simulink model "Filtri_Dinamici"  (R2022b)
settings: Solver=ode45  StartTime=0.0  StopTime=time_max  RelTol=1e-3
values from neighbouring files (symbols this model uses):
  b_omega_hat0 = [0;0;0]    [Main_Articolo.m]
  bias_accel = [bias_a_x; bias_a_y; bias_a_z]    [Main_Articolo.m]
  bias_gyro = [bias_gyro_x; bias_gyro_y; bias_gyro_z]    [Main_Articolo.m]    (also in Plot_Filtri_Din.m = out.bias_gyro.Data)
  bias_magn = [bias_magn_x; bias_magn_y; bias_magn_z]    [Main_Articolo.m]
  Delta = 0.03    [Main_Articolo.m]
  dev_std_a_x = 0.0248    [Main_Articolo.m]
  dev_std_a_y = 0.0248    [Main_Articolo.m]
  dev_std_a_z = 0.0203    [Main_Articolo.m]
  dev_std_gyro_x = 2.653*10^(-3)    (= 0.002653)    [Main_Articolo.m]
  dev_std_gyro_y = 2.653*10^(-3)    (= 0.002653)    [Main_Articolo.m]
  dev_std_gyro_z = 3.159*10^(-3)    (= 0.003159)    [Main_Articolo.m]
  dev_std_magn_x = 0.01    [Main_Articolo.m]
  dev_std_magn_y = 0.015    [Main_Articolo.m]
  dev_std_magn_z = 0.0175    [Main_Articolo.m]
  dt = 0.01    [Main_Articolo.m]
  g = 9.81    [Main_Articolo.m]
  k1 = 1    [Main_Articolo.m]
  k1_CO = 1    [Main_Articolo.m]
  k1_MS = 1    [Main_Articolo.m]
  k2 = 0.2    [Main_Articolo.m]
  k2_CO = 0.2    [Main_Articolo.m]
  k2_MS = 0.2    [Main_Articolo.m]
  k3_CO = k1_CO/32    (= 0.03125)    [Main_Articolo.m]
  k4_CO = k2_CO/32    (= 0.00625)    [Main_Articolo.m]
  k_B = 1/32    (= 0.03125)    [Main_Articolo.m]
  k_B_MS = 1/32    (= 0.03125)    [Main_Articolo.m]
  kB_CO = 16    [Main_Articolo.m]
  m_I = [m_i_x; 0; m_i_z]    [Main_Articolo.m]
  Omega11 = 0.075    [Main_Articolo.m]
  Omega12 = 0.045    [Main_Articolo.m]
  Omega13 = 0.02    [Main_Articolo.m]
  Omega21 = 0.085    [Main_Articolo.m]
  Omega22 = -0.03    [Main_Articolo.m]
  Omega23 = 0.015    [Main_Articolo.m]
  Omega31 = 0.1    [Main_Articolo.m]
  Omega32 = 0.036    [Main_Articolo.m]
  Omega33 = -0.025    [Main_Articolo.m]
  Phi1 = 40*pi/180    (= 0.698131700798)    [Main_Articolo.m]
  Phi2 = 20*pi/180    (= 0.349065850399)    [Main_Articolo.m]
  Phi3 = 2*pi/180    (= 0.0349065850399)    [Main_Articolo.m]
  phi_0 = 15*pi/180    (= 0.261799387799)    [Main_Articolo.m]
  pos_0 = [x_0; y_0; z_0]    [Main_Articolo.m]
  Psi1 = 160*pi/180    (= 2.79252680319)    [Main_Articolo.m]
  Psi2 = 35*pi/180    (= 0.610865238198)    [Main_Articolo.m]
  Psi3 = 5*pi/180    (= 0.0872664625997)    [Main_Articolo.m]
  psi_0 = pi/4    (= 0.785398163397)    [Main_Articolo.m]
  R0 = eye(3)    [Main_Articolo.m]
  R_0_esatta = [cos(theta_0)*cos(psi_0),  -cos(phi_0)*sin(psi_0) + cos(psi_0)*sin(phi_0)*sin(theta_0),   sin(phi_0)*sin(psi_0) + cos(psi_0)*cos(phi_0)*sin(theta_0) ... (first row only)    [Main_Articolo.m]
  rumori_bias = 1    [Main_Articolo.m]
  Theta1 = 50*pi/180    (= 0.872664625997)    [Main_Articolo.m]
  Theta2 = 12*pi/180    (= 0.209439510239)    [Main_Articolo.m]
  Theta3 = 3*pi/180    (= 0.0523598775598)    [Main_Articolo.m]
  theta_0 = 10*pi/180    (= 0.174532925199)    [Main_Articolo.m]
  vel_0 = [dx_0; dy_0; dz_0]    [Main_Articolo.m]
  w_11 = 2*pi/30    (= 0.209439510239)    [Main_Articolo.m]
  w_12 = 2*pi/12    (= 0.523598775598)    [Main_Articolo.m]
  w_13 = 2*pi/4    (= 1.57079632679)    [Main_Articolo.m]
  w_21 = 2*pi/25    (= 0.251327412287)    [Main_Articolo.m]
  w_22 = 2*pi/18    (= 0.349065850399)    [Main_Articolo.m]
  w_23 = 2*pi/3    (= 2.09439510239)    [Main_Articolo.m]
  w_31 = 2*pi/20    (= 0.314159265359)    [Main_Articolo.m]
  w_32 = 2*pi/10    (= 0.628318530718)    [Main_Articolo.m]
  w_33 = 2*pi/2    (= 3.14159265359)    [Main_Articolo.m]
  w_phi1 = 2*pi/27    (= 0.232710566933)    [Main_Articolo.m]
  w_phi2 = 2*pi/18    (= 0.349065850399)    [Main_Articolo.m]
  w_phi3 = 2*pi/3    (= 2.09439510239)    [Main_Articolo.m]
  w_psi1 = 2*pi/30    (= 0.209439510239)    [Main_Articolo.m]
  w_psi2 = 2*pi/15    (= 0.418879020479)    [Main_Articolo.m]
  w_psi3 = 2*pi/4    (= 1.57079632679)    [Main_Articolo.m]
  w_theta1 = 2*pi/23    (= 0.273181969877)    [Main_Articolo.m]
  w_theta2 = 2*pi/12    (= 0.523598775598)    [Main_Articolo.m]
  w_theta3 = 2*pi/3.5    (= 1.79519580205)    [Main_Articolo.m]
  x_Mahony0 = [phi_0; theta_0; psi_0]    [Main_Articolo.m]
settings Model: Creator=paoga  LastModifiedBy=paoga

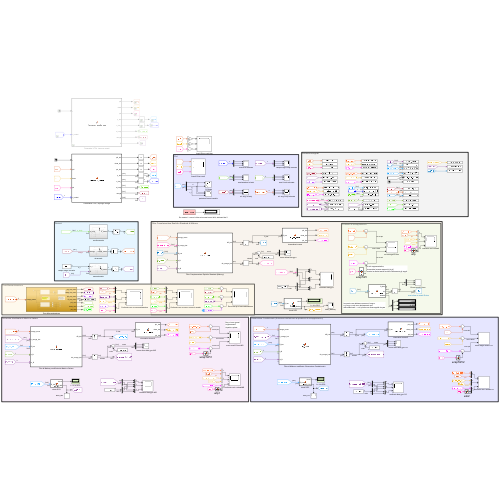
[thumbnail: Simulink's stored preview of the top-level diagram]
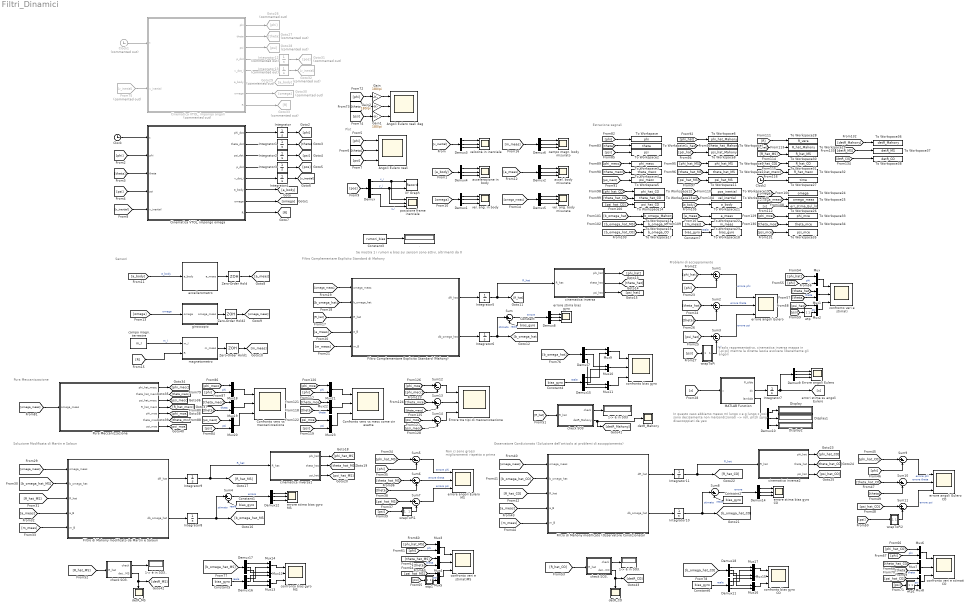
== system Filtri_Dinamici ==
  note: Estrazione segnali
  note: Pura Meccanizzazione
  note: è solo rappresentativo,
      | cinematica inversa mappa in [-pi;pi]
      | mentre la diretta lascia evolvere liberamente gli angoli
  note: Se mostra 1 i rumori e bias sui sensori sono attivi, altrimenti da 0
  note: Osservatore Condizionato (Soluzione dell'articolo ai problemi di accoppiamento)
  note: Non ci sono grossi
      | miglioramenti
      | rispetto a prima
  note: Soluzione Modificata di Martin e Salaun
  note: Problemi di accoppiamento
  note: In questo caso abbiamo messo mI lungo x
      | e g lungo z così sono decisamente non
      | malcondizionati --> roll, pitch sono disaccoppiati da yaw
  note: Filtro Complementare Esplicito Standard di Mahony
  note: Sensori
  note: Plot
  . : Display
  1-> è in SO3 : Display
  1-> è in SO3. : Display
  1-> è in SO3.. : Display
  Angoli Eulero reali : Scope  NumInputPorts=3
  Angoli Eulero reali deg : Scope  NumInputPorts=3
  "Cinematica VTOL, impongo angoli" : MATLAB Function  Commented=on  TreatAsAtomicUnit=on
  "Cinematica VTOL, impongo omega" : MATLAB Function  TreatAsAtomicUnit=on
  Clock : Clock
  Clock1 : Clock  Commented=on
  Clock2 : Clock
  Confronto vero vs mecc come cin esatta : Scope  NumInputPorts=3
  Confronto vero vs meccanizzazione : Scope  NumInputPorts=3
  Constant{,1..2,4..7} (7 alike) : Constant  Value=bias_gyro
  Constant3 : Constant  Value=rumori_bias
  Demux{,1..12,14..18} (18 alike) : Demux  Outputs=3
  Display : Display
  Display1 : Display
  Display2 : Display
  Errore angoli Eulero : Scope  NumInputPorts=3
  Errore tra tipi di meccanizzazione : Scope  NumInputPorts=3
  Filtro Complementare Esplicito Standard (Mahony) : MATLAB Function  TreatAsAtomicUnit=on
  Filtro di Mahony modificato (Osservatore Condizionato) : MATLAB Function  TreatAsAtomicUnit=on
  Filtro di Mahony modificato da Martin e Salaun : MATLAB Function  TreatAsAtomicUnit=on
  From75 : From  Commented=on  GotoTag=v_inertial
  Gain : Gain  Gain=180/pi
  Gain1 : Gain  Gain=180/pi
  Gain2 : Gain  Gain=180/pi
  Goto26 : Goto  Commented=on  GotoTag=phi
  Goto27 : Goto  Commented=on  GotoTag=theta
  Goto28 : Goto  Commented=on  GotoTag=psi
  Goto29 : Goto  Commented=on  GotoTag=a_body
  Goto30 : Goto  Commented=on  GotoTag=omega
  Goto31 : Goto  Commented=on  GotoTag=pos
  Goto32 : Goto  Commented=on  GotoTag=v_inertial
  Goto33 : Goto  Commented=on  GotoTag=R
  Integrator : Integrator  InitialCondition=phi_0
  Integrator1 : Integrator  InitialCondition=theta_0
  Integrator10 : Integrator  InitialCondition=b_omega_hat0
  Integrator11 : Integrator  InitialCondition=R0
  Integrator12 : Integrator  Commented=on  InitialCondition=pos_0
  Integrator13 : Integrator  Commented=on  InitialCondition=vel_0
  Integrator2 : Integrator  InitialCondition=psi_0
  Integrator3 : Integrator  InitialCondition=pos_0
  Integrator4 : Integrator  InitialCondition=vel_0
  Integrator5 : Integrator  InitialCondition=R0
  Integrator6 : Integrator  InitialCondition=b_omega_hat0
  Integrator7 : Integrator  InitialCondition=x_Mahony0
  Integrator8 : Integrator  InitialCondition=b_omega_hat0
  Integrator9 : Integrator  InitialCondition=R0
  MATLAB Function : MATLAB Function  TreatAsAtomicUnit=on
  Mux{,1..23} (24 alike) : Mux  Inputs=2
  Pura Meccanizzazione : Subsystem
  Sum{,1..14} (15 alike) : Sum  Inputs=|+-
  To Workspace : ToWorkspace  VariableName=phi  SaveFormat=Timeseries  SampleTime=-1
  To Workspace1 : ToWorkspace  VariableName=theta  SaveFormat=Timeseries  SampleTime=-1
  To Workspace10 : ToWorkspace  VariableName=theta_hat_MS  SaveFormat=Timeseries  SampleTime=-1
  To Workspace11 : ToWorkspace  VariableName=psi_hat_MS  SaveFormat=Timeseries  SampleTime=-1
  To Workspace12 : ToWorkspace  VariableName=phi_hat_CO  SaveFormat=Timeseries  SampleTime=-1
  To Workspace13 : ToWorkspace  VariableName=theta_hat_CO  SaveFormat=Timeseries  SampleTime=-1
  To Workspace14 : ToWorkspace  VariableName=psi_hat_CO  SaveFormat=Timeseries  SampleTime=-1
  To Workspace15 : ToWorkspace  VariableName=b_omega_Mahony  SaveFormat=Timeseries  SampleTime=-1
  To Workspace16 : ToWorkspace  VariableName=b_omega_MS  SaveFormat=Timeseries  SampleTime=-1
  To Workspace17 : ToWorkspace  VariableName=b_omega_CO  SaveFormat=Timeseries  SampleTime=-1
  To Workspace18 : ToWorkspace  VariableName=bias_gyro  SaveFormat=Timeseries  SampleTime=-1
  To Workspace19 : ToWorkspace  VariableName=pos_inertial  SaveFormat=Timeseries  SampleTime=-1
  To Workspace2 : ToWorkspace  VariableName=psi  SaveFormat=Timeseries  SampleTime=-1
  To Workspace20 : ToWorkspace  VariableName=vel_inertial  SaveFormat=Timeseries  SampleTime=-1
  To Workspace21 : ToWorkspace  VariableName=a_body  SaveFormat=Timeseries  SampleTime=-1
  To Workspace22 : ToWorkspace  VariableName=a_meas  SaveFormat=Timeseries  SampleTime=-1
  To Workspace23 : ToWorkspace  VariableName=m_meas  SaveFormat=Timeseries  SampleTime=-1
  To Workspace24 : ToWorkspace  VariableName=omega  SaveFormat=Timeseries  SampleTime=-1
  To Workspace25 : ToWorkspace  VariableName=omega_meas  SaveFormat=Timeseries  SampleTime=-1
  To Workspace26 : ToWorkspace  VariableName=err_stima_Eul_lin  SaveFormat=Timeseries  SampleTime=-1
  To Workspace27 : ToWorkspace  VariableName=time  SampleTime=-1
  To Workspace28 : ToWorkspace  VariableName=R_vera  SampleTime=-1
  To Workspace29 : ToWorkspace  VariableName=R_hat_Mahony  SampleTime=-1
  To Workspace3 : ToWorkspace  VariableName=phi_mecc  SaveFormat=Timeseries  SampleTime=-1
  To Workspace30 : ToWorkspace  VariableName=R_hat_MS  SampleTime=-1
  To Workspace31 : ToWorkspace  VariableName=R_hat_CO  SampleTime=-1
  To Workspace32 : ToWorkspace  VariableName=R_hat_mecc  SampleTime=-1
  To Workspace33 : ToWorkspace  VariableName=phi_mce  SaveFormat=Timeseries  SampleTime=-1
  To Workspace34 : ToWorkspace  VariableName=theta_mce  SaveFormat=Timeseries  SampleTime=-1
  To Workspace35 : ToWorkspace  VariableName=psi_mce  SaveFormat=Timeseries  SampleTime=-1
  To Workspace36 : ToWorkspace  VariableName=detR_Mahony  SaveFormat=Timeseries  SampleTime=-1
  To Workspace37 : ToWorkspace  VariableName=detR_MS  SaveFormat=Timeseries  SampleTime=-1
  To Workspace38 : ToWorkspace  VariableName=detR_CO  SaveFormat=Timeseries  SampleTime=-1
  To Workspace4 : ToWorkspace  VariableName=theta_mecc  SaveFormat=Timeseries  SampleTime=-1
  To Workspace5 : ToWorkspace  VariableName=psi_mecc  SaveFormat=Timeseries  SampleTime=-1
  To Workspace6 : ToWorkspace  VariableName=phi_hat_Mahony  SaveFormat=Timeseries  SampleTime=-1
  To Workspace7 : ToWorkspace  VariableName=theta_hat_Mahony  SaveFormat=Timeseries  SampleTime=-1
  To Workspace8 : ToWorkspace  VariableName=psi_hat_Mahony  SaveFormat=Timeseries  SampleTime=-1
  To Workspace9 : ToWorkspace  VariableName=phi_hat_MS  SaveFormat=Timeseries  SampleTime=-1
  XY Graph : Record  FileSettingsInternal="{\"entries\":[{\"content\":{\"excelSettings\":{\"content\":{},\"type\":\"Streamout.ExcelSettings\"}},\"type\":\"Streamout.FileSettingStorage\",\"uuid\":\"1bb055d0-a70c-4173-8516-ac4b5ad9ec40\"}],\"packageUris\":[\"http://schema.mathworks.com/mf0/streamout_blocks/R2020a\"],\"version\":\"1.0\"}"  Layout=[1 1]  SignalsInternal="{\"entries\":[{\"content\":{\"signals\":[{\"content\":{\"blockPath\":[\"Filtri_Dinamici/XY Graph\"],\"channel\":[],\"dimensions\":[1,1],\"domain\":\"Filtri_Dinamici/XY Graph\",\"lineColor\":\"#a2142f\",\"plots\":[1],\"port\":1,\"sid\":[\"\"],\"signalID\":2126,\"signalName\":\"x_i\"},\"type\":\"RecordBlkView.Signal\",\"uuid\":\"c40f1304-f7aa-464d-a0d5-21e988c50381\"},{\"content\":{\"blockPath\":[\"Filtri_Dinamici/XY Graph\"],\"channel\":[],\"dimensions\":[1,1],\"domain\":\"Filtri_Dinamici/XY Graph\",\"lineColor\":\"#139fff\",\"plots\":[1],\"port\":2,\"sid\":[\"\"],\"signalID\":2130,\"signalName\":\"y_i\"},\"type\":\"RecordBlkView.Signal\",\"uuid\":\"5add5732-de02-4d21-bdf5-598b3397d51e\"}]},\"type\":\"RecordBlkView.InputSignals\",\"uuid\":\"cac5dfdf-c4f8-45da-884d-dcbd0f080275\"}],\"packageUris\":[\"http://schema.mathworks.com/mf0/streamout_blocks/R2020a\"],\"version\":\"1.0\"}"  VisualizationBindings="{\"xyplotplugin\":{\"info\":[{\"series\":[{\"bindingParametersList\":[{\"parameter\":\"X-Axis\",\"signalID\":2126,\"signalName\":\"x_i\"},{\"parameter\":\"Y-Axis\",\"signalID\":2130,\"signalName\":\"y_i\"}],\"seriesID\":17403}],\"subplotID\":1}]}}"  CompatibilityTag=XY
  Zero-Order Hold : ZeroOrderHold  SampleTime=dt
  Zero-Order Hold1 : ZeroOrderHold  SampleTime=dt
  Zero-Order Hold2 : ZeroOrderHold  SampleTime=dt
  accel. body misurata : Scope  NumInputPorts=3
  accelerazione in body : Scope  NumInputPorts=3
  accellerometro : Subsystem
  campo magn. body misurato : Scope  NumInputPorts=3
  campo magn. terrestre : Constant  Value=m_I
  check SO3 : MATLAB Function  TreatAsAtomicUnit=on
  check SO3, : MATLAB Function  TreatAsAtomicUnit=on
  check SO3. : MATLAB Function  TreatAsAtomicUnit=on
  cinematica inversa : MATLAB Function  TreatAsAtomicUnit=on
  cinematica inversa1 : MATLAB Function  TreatAsAtomicUnit=on
  cinematica inversa2 : MATLAB Function  TreatAsAtomicUnit=on
  "confronto bias gyro " : Scope  NumInputPorts=3
  confronto bias gyro CO : Scope  NumInputPorts=3
  confronto bias gyro MS : Scope  NumInputPorts=3
  confronto veri e stimati : Scope  NumInputPorts=3
  confronto veri e stimati CO : Scope  NumInputPorts=3
  confronto veri e stimatiMS : Scope  NumInputPorts=3
  detR_CO : Scope
  detR_MS : Scope
  detR_Mahony : Scope
  errore angoli Eulero : Scope  NumInputPorts=3
  errore angoli Eulero CO : Scope  NumInputPorts=3
  errore angoli Eulero MS : Scope  NumInputPorts=3
  errore stima bias gyro : Scope  NumInputPorts=3
  errore stima bias gyro CO : Scope  NumInputPorts=3
  errore stima bias gyro MS : Scope  NumInputPorts=3
  giroscopio : Subsystem
  magnetometro : Subsystem
  posizione frame inerziale : Scope  NumInputPorts=3
  vel. ang. body misurata : Scope  NumInputPorts=3
  vel. ang. in body : Scope  NumInputPorts=3
  velocità in inerziale : Scope  NumInputPorts=3
  wrapToPi : MATLAB Function  TreatAsAtomicUnit=on
  wrapToPi1 : MATLAB Function  TreatAsAtomicUnit=on
  wrapToPi2 : MATLAB Function  TreatAsAtomicUnit=on
  wtp : MATLAB Function  TreatAsAtomicUnit=on
  wtp1 : MATLAB Function  TreatAsAtomicUnit=on
  wtp2 : MATLAB Function  TreatAsAtomicUnit=on
  wires:
  Clock/1 -> "Cinematica VTOL, impongo omega"/1(t)
  "Cinematica VTOL, impongo omega"/1(phi_dot) -> Integrator/1
  Integrator/1 -> [phi]
  [phi] -> "Cinematica VTOL, impongo omega"/2(phi)
  "Cinematica VTOL, impongo omega"/2(theta_dot) -> Integrator1/1
  "Cinematica VTOL, impongo omega"/3(psi_dot) -> Integrator2/1
  Integrator1/1 -> [theta]
  Integrator2/1 -> [psi]
  [theta] -> "Cinematica VTOL, impongo omega"/3(theta)
  [psi] -> "Cinematica VTOL, impongo omega"/4(psi)
  [phi] -> Angoli Eulero reali/1
  [theta] -> Angoli Eulero reali/2
  [psi] -> Angoli Eulero reali/3
  "Cinematica VTOL, impongo omega"/4(p_dot) -> Integrator3/1
  Integrator3/1 -> [pos]
  "Cinematica VTOL, impongo omega"/5(v_dot_i) -> Integrator4/1
  [v_inertial] -> "Cinematica VTOL, impongo omega"/5(v_inertial)
  [pos] -> Demux/1
  Demux/1 -> XY Graph/1, posizione frame inerziale/1  "x_i"
  Demux/2 -> XY Graph/2, posizione frame inerziale/2  "y_i"
  Demux/3 -> posizione frame inerziale/3  "z_i"
  Demux3/1 -> velocità in inerziale/1
  Demux3/3 -> velocità in inerziale/3
  Demux3/2 -> velocità in inerziale/2
  Demux4/1 -> accelerazione in body/1
  Demux4/3 -> accelerazione in body/3
  Demux4/2 -> accelerazione in body/2
  [v_inertial] -> Demux3/1
  Integrator4/1 -> [v_inertial]
  "Cinematica VTOL, impongo omega"/6(a_body) -> [a_body]
  [a_body] -> Demux4/1
  "Cinematica VTOL, impongo omega"/7(omega) -> [omega]
  [omega] -> Demux1/1
  Demux1/2 -> vel. ang. in body/2
  Demux1/1 -> vel. ang. in body/1
  Demux1/3 -> vel. ang. in body/3
  "Cinematica VTOL, impongo omega"/8(R) -> [R]
  [a_body] -> accellerometro/1(a_body)  "a_body"
  accellerometro/1(a_meas) -> Zero-Order Hold/1
  [a_meas] -> Demux2/1
  Demux2/1 -> accel. body misurata/1
  Demux2/2 -> accel. body misurata/2
  Demux2/3 -> accel. body misurata/3
  [omega] -> giroscopio/1(omega)  "omega"
  giroscopio/1(omega_meas) -> Zero-Order Hold2/1
  [omega_meas] -> Demux5/1
  Demux5/1 -> vel. ang. body misurata/1
  Demux5/2 -> vel. ang. body misurata/2
  Demux5/3 -> vel. ang. body misurata/3
  campo magn. terrestre/1 -> magnetometro/1(m_I)  "m_I"
  [R] -> magnetometro/2(R)
  magnetometro/1(m_meas) -> Zero-Order Hold1/1
  [m_meas] -> Demux6/1
  Demux6/2 -> campo magn. body misurato/2
  Demux6/3 -> campo magn. body misurato/3
  Demux6/1 -> campo magn. body misurato/1
  Filtro Complementare Esplicito Standard (Mahony)/1(dR_hat) -> Integrator5/1
  Integrator5/1 -> cinematica inversa/1(R_hat), [R_hat]  "R_hat"
  [R_hat] -> Filtro Complementare Esplicito Standard (Mahony)/3(R_hat)
  Filtro Complementare Esplicito Standard (Mahony)/2(db_omega_hat) -> Integrator6/1
  Integrator6/1 -> [b_omega_hat], Sum/1  "stimato"
  [b_omega_hat] -> Filtro Complementare Esplicito Standard (Mahony)/2(b_omega_hat)
  [omega_meas] -> Filtro Complementare Esplicito Standard (Mahony)/1(omega_meas)
  [a_meas] -> Filtro Complementare Esplicito Standard (Mahony)/4(a_B)
  [m_meas] -> Filtro Complementare Esplicito Standard (Mahony)/5(m_B)
  Constant/1 -> Sum/2  "reale"
  Sum/1 -> Demux8/1  "errore"
  Demux8/1 -> errore stima bias gyro/1
  Demux8/2 -> errore stima bias gyro/2
  Demux8/3 -> errore stima bias gyro/3
  cinematica inversa/1(phi_hat) -> [phi_hat]
  cinematica inversa/2(theta_hat) -> [theta_hat]
  cinematica inversa/3(psi_hat) -> [psi_hat]
  [phi_hat] -> Sum1/1
  [phi] -> Sum1/2
  Sum1/1 -> errore angoli Eulero/1  "errore phi"
  [psi_hat] -> Sum3/1
  [theta_hat] -> Sum2/1
  [theta] -> Sum2/2
  Sum2/1 -> errore angoli Eulero/2  "errore theta"
  Sum3/1 -> errore angoli Eulero/3  "errore psi"
  [psi] -> wrapToPi/1(u)
  Zero-Order Hold/1 -> [a_meas]
  Zero-Order Hold2/1 -> [omega_meas]
  Zero-Order Hold1/1 -> [m_meas]
  MATLAB Function/2(dx) -> Integrator7/1
  Integrator7/1 -> [x], Demux9/1
  [x] -> MATLAB Function/1(x)
  Demux9/3 -> Errore angoli Eulero/3
  Demux9/2 -> Errore angoli Eulero/2
  Demux9/1 -> Errore angoli Eulero/1
  MATLAB Function/3(lambda) -> Demux10/1
  Demux10/1 -> Display/1
  Demux10/2 -> Display1/1
  Demux10/3 -> Display2/1
  [omega_meas] -> Filtro di Mahony modificato da Martin e Salaun/1(omega_meas)
  Filtro di Mahony modificato da Martin e Salaun/2(db_omega_hat) -> Integrator8/1
  [b_omega_hat_MS] -> Filtro di Mahony modificato da Martin e Salaun/2(b_omega_hat)
  Filtro di Mahony modificato da Martin e Salaun/1(dR_hat) -> Integrator9/1
  [R_hat_MS] -> Filtro di Mahony modificato da Martin e Salaun/3(R_hat)
  Demux12/3 -> errore stima bias gyro MS/3
  Demux12/1 -> errore stima bias gyro MS/1
  Constant1/1 -> Sum4/2  "reale"
  Integrator8/1 -> Sum4/1, [b_omega_hat_MS]  "stimato"
  Demux12/2 -> errore stima bias gyro MS/2
  Sum4/1 -> Demux12/1  "errore"
  cinematica inversa1/2(theta_hat) -> [theta_hat_MS]
  cinematica inversa1/1(phi_hat) -> [phi_hat_MS]
  cinematica inversa1/3(psi_hat) -> [psi_hat_MS]
  [a_meas] -> Filtro di Mahony modificato da Martin e Salaun/4(a_B)
  [m_meas] -> Filtro di Mahony modificato da Martin e Salaun/5(m_B)
  Sum6/1 -> errore angoli Eulero MS/2  "errore theta"
  [phi_hat_MS] -> Sum5/1
  Sum7/1 -> errore angoli Eulero MS/3  "errore psi"
  [theta_hat_MS] -> Sum6/1
  [psi] -> wrapToPi1/1(u)
  [theta] -> Sum6/2
  Sum5/1 -> errore angoli Eulero MS/1  "errore phi"
  [phi] -> Sum5/2
  [psi_hat_MS] -> Sum7/1
  [omega_meas] -> Filtro di Mahony modificato (Osservatore Condizionato)/1(omega_meas)
  [b_omega_hat_CO] -> Filtro di Mahony modificato (Osservatore Condizionato)/2(b_omega_hat)
  [R_hat_CO] -> Filtro di Mahony modificato (Osservatore Condizionato)/3(R_hat)
  [a_meas] -> Filtro di Mahony modificato (Osservatore Condizionato)/4(a_B)
  [m_meas] -> Filtro di Mahony modificato (Osservatore Condizionato)/5(m_B)
  Demux14/2 -> errore stima bias gyro CO/2
  Sum8/1 -> Demux14/1  "errore"
  Demux14/3 -> errore stima bias gyro CO/3
  Filtro di Mahony modificato (Osservatore Condizionato)/1(dR_hat) -> Integrator11/1
  Demux14/1 -> errore stima bias gyro CO/1
  cinematica inversa2/2(theta_hat) -> [theta_hat_CO]
  [psi_hat_CO] -> Sum11/1
  [phi_hat_CO] -> Sum9/1
  Sum11/1 -> errore angoli Eulero CO/3  "errore psi"
  [theta] -> Sum10/2
  [psi] -> wrapToPi2/1(u)
  cinematica inversa2/1(phi_hat) -> [phi_hat_CO]
  [theta_hat_CO] -> Sum10/1
  cinematica inversa2/3(psi_hat) -> [psi_hat_CO]
  Sum10/1 -> errore angoli Eulero CO/2  "errore theta"
  [phi] -> Sum9/2
  Constant2/1 -> Sum8/2  "reale"
  Sum9/1 -> errore angoli Eulero CO/1  "errore phi"
  Integrator10/1 -> Sum8/1, [b_omega_hat_CO]  "stimato"
  Filtro di Mahony modificato (Osservatore Condizionato)/2(db_omega_hat) -> Integrator10/1
  Constant3/1 -> ./1
  check SO3/1(check) -> 1-> è in SO3/1
  Integrator9/1 -> cinematica inversa1/1(R_hat), [R_hat_MS]  "R_hat"
  check SO3./1(check) -> 1-> è in SO3../1
  check SO3,/1(check) -> 1-> è in SO3./1
  Integrator11/1 -> cinematica inversa2/1(R_hat), [R_hat_CO]  "R_hat"
  [R_hat] -> check SO3/1(R_hat)
  [R_hat_MS] -> check SO3./1(R_hat)
  [R_hat_CO] -> check SO3,/1(R_hat)
  wrapToPi/1(y) -> Sum3/2  "psi"
  wrapToPi1/1(y) -> Sum7/2
  wrapToPi2/1(y) -> Sum11/2
  [phi_hat] -> Mux/1
  [phi] -> Mux/2  "phi"
  [theta_hat] -> Mux1/1
  [theta] -> Mux1/2  "theta"
  [psi_hat] -> Mux2/1
  [psi] -> wtp/1(u)
  wtp/1(y) -> Mux2/2  "psi"
  Mux/1 -> confronto veri e stimati/1
  Mux1/1 -> confronto veri e stimati/2
  Mux2/1 -> confronto veri e stimati/3
  Mux4/1 -> confronto veri e stimatiMS/2
  Mux3/1 -> confronto veri e stimatiMS/1
  [theta] -> Mux4/2  "theta"
  [phi] -> Mux3/2  "phi"
  Mux5/1 -> confronto veri e stimatiMS/3
  [theta_hat_MS] -> Mux4/1
  [psi] -> wtp1/1(u)
  [psi_hat_MS] -> Mux5/1
  wtp1/1(y) -> Mux5/2  "psi"
  [phi_hat_MS] -> Mux3/1
  Mux7/1 -> confronto veri e stimati CO/2
  Mux6/1 -> confronto veri e stimati CO/1
  [theta] -> Mux7/2  "theta"
  [phi] -> Mux6/2  "phi"
  Mux8/1 -> confronto veri e stimati CO/3
  [theta_hat_CO] -> Mux7/1
  [psi] -> wtp2/1(u)
  [psi_hat_CO] -> Mux8/1
  wtp2/1(y) -> Mux8/2  "psi"
  [phi_hat_CO] -> Mux6/1
  [psi] -> Gain1/1
  [phi] -> Gain/1
  [theta] -> Gain2/1
  Gain/1 -> Angoli Eulero reali deg/1
  Gain2/1 -> Angoli Eulero reali deg/2
  Gain1/1 -> Angoli Eulero reali deg/3
  Clock1/1 -> "Cinematica VTOL, impongo angoli"/1(t)
  "Cinematica VTOL, impongo angoli"/1(phi) -> Goto26/1
  "Cinematica VTOL, impongo angoli"/2(theta) -> Goto27/1
  "Cinematica VTOL, impongo angoli"/3(psi) -> Goto28/1
  "Cinematica VTOL, impongo angoli"/4(p_dot) -> Integrator12/1
  "Cinematica VTOL, impongo angoli"/8(R) -> Goto33/1
  Integrator12/1 -> Goto31/1
  "Cinematica VTOL, impongo angoli"/7(omega) -> Goto30/1
  "Cinematica VTOL, impongo angoli"/5(v_dot_i) -> Integrator13/1
  Integrator13/1 -> Goto32/1
  "Cinematica VTOL, impongo angoli"/6(a_body) -> Goto29/1
  From75/1 -> "Cinematica VTOL, impongo angoli"/2(v_inertial)
  [b_omega_hat] -> Demux7/1
  Constant4/1 -> Demux15/1  "reale"
  Mux9/1 -> "confronto bias gyro "/1
  Mux10/1 -> "confronto bias gyro "/2
  Mux11/1 -> "confronto bias gyro "/3
  Demux7/1 -> Mux9/1
  Demux15/1 -> Mux9/2
  Demux7/2 -> Mux10/1
  Demux15/2 -> Mux10/2
  Demux7/3 -> Mux11/1
  Demux15/3 -> Mux11/2
  Constant5/1 -> Demux16/1  "reale"
  Demux16/3 -> Mux13/2
  Demux17/3 -> Mux13/1
  Mux13/1 -> confronto bias gyro MS/3
  Demux16/1 -> Mux14/2
  Mux12/1 -> confronto bias gyro MS/2
  [b_omega_hat_MS] -> Demux17/1
  Mux14/1 -> confronto bias gyro MS/1
  Demux17/1 -> Mux14/1
  Demux16/2 -> Mux12/2
  Demux17/2 -> Mux12/1
  Constant6/1 -> Demux11/1  "reale"
  Demux11/3 -> Mux16/2
  Demux18/3 -> Mux16/1
  Mux16/1 -> confronto bias gyro CO/3
  Demux11/1 -> Mux17/2
  Mux15/1 -> confronto bias gyro CO/2
  [b_omega_hat_CO] -> Demux18/1
  Mux17/1 -> confronto bias gyro CO/1
  Demux18/1 -> Mux17/1
  Demux11/2 -> Mux15/2
  Demux18/2 -> Mux15/1
  [omega_meas] -> Pura Meccanizzazione/1(omega_meas)
  Mux20/1 -> Confronto vero vs meccanizzazione/3
  [phi] -> Mux18/2  "phi"
  Mux19/1 -> Confronto vero vs meccanizzazione/2
  [psi] -> Mux20/2  "psi"
  [theta] -> Mux19/2  "theta"
  Mux18/1 -> Confronto vero vs meccanizzazione/1
  [phi] -> To Workspace/1
  [theta] -> To Workspace1/1
  [psi] -> To Workspace2/1
  Pura Meccanizzazione/1(phi_hat_mecc) -> [phi_mecc]
  Pura Meccanizzazione/2(theta_hat_mecc) -> [theta_mecc]
  Pura Meccanizzazione/3(psi_hat_mecc) -> [psi_mecc]
  [phi_mecc] -> Mux18/1
  [theta_mecc] -> Mux19/1
  [psi_mecc] -> Mux20/1
  [theta_mecc] -> To Workspace4/1
  [psi_mecc] -> To Workspace5/1
  [phi_mecc] -> To Workspace3/1
  [theta_hat] -> To Workspace7/1
  [phi_hat] -> To Workspace6/1
  [psi_hat] -> To Workspace8/1
  [phi_hat_MS] -> To Workspace9/1
  [theta_hat_MS] -> To Workspace10/1
  [psi_hat_MS] -> To Workspace11/1
  [phi_hat_CO] -> To Workspace12/1
  [theta_hat_CO] -> To Workspace13/1
  [psi_hat_CO] -> To Workspace14/1
  [b_omega_hat] -> To Workspace15/1
  [b_omega_hat_MS] -> To Workspace16/1
  [b_omega_hat_CO] -> To Workspace17/1
  Constant7/1 -> To Workspace18/1  "reale"
  [pos] -> To Workspace19/1
  [v_inertial] -> To Workspace20/1
  [a_body] -> To Workspace21/1
  [a_meas] -> To Workspace22/1
  [m_meas] -> To Workspace23/1
  [omega] -> To Workspace24/1
  [omega_meas] -> To Workspace25/1
  [x] -> To Workspace26/1
  Clock2/1 -> To Workspace27/1
  [R] -> To Workspace28/1
  [R_hat] -> To Workspace29/1
  [R_hat_MS] -> To Workspace30/1
  [R_hat_CO] -> To Workspace31/1
  Pura Meccanizzazione/4(R_hat_mecc) -> [R_hat_mecc]
  [R_hat_mecc] -> To Workspace32/1
  Pura Meccanizzazione/5(phi_mce) -> [phi_mce]
  Pura Meccanizzazione/6(theta_mce) -> [theta_mce]
  Pura Meccanizzazione/7(psi_mce) -> [psi_mce]
  [phi_mce] -> Mux21/1
  Mux21/1 -> Confronto vero vs mecc come cin esatta/1
  [theta_mce] -> Mux22/1
  [theta] -> Mux22/2  "theta"
  Mux22/1 -> Confronto vero vs mecc come cin esatta/2
  [psi] -> Mux23/2  "psi"
  [phi] -> Mux21/2  "phi"
  Mux23/1 -> Confronto vero vs mecc come cin esatta/3
  [psi_mce] -> Mux23/1
  [phi_mce] -> Sum12/1
  [theta_mce] -> Sum13/1
  [theta_mecc] -> Sum13/2
  [psi_mecc] -> Sum14/2
  [phi_mecc] -> Sum12/2
  [psi_mce] -> Sum14/1
  Sum12/1 -> Errore tra tipi di meccanizzazione/1
  Sum13/1 -> Errore tra tipi di meccanizzazione/2
  Sum14/1 -> Errore tra tipi di meccanizzazione/3
  [phi_mce] -> To Workspace33/1
  [theta_mce] -> To Workspace34/1
  [psi_mce] -> To Workspace35/1
  check SO3/2(detR_Mahony) -> detR_Mahony/1, [detR_Mahony]
  [detR_Mahony] -> To Workspace36/1
  check SO3./2(detR_MS) -> [detR_MS], detR_MS/1
  check SO3,/2(detR_CO) -> [detR_CO], detR_CO/1
  [detR_MS] -> To Workspace37/1
  [detR_CO] -> To Workspace38/1

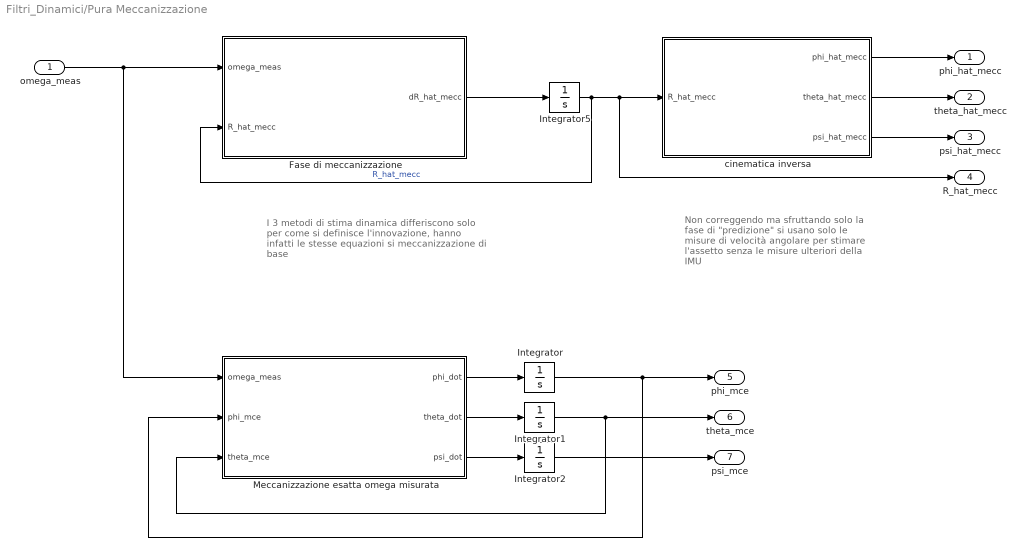
== system Filtri_Dinamici/Pura Meccanizzazione ==
  note: Non correggendo ma sfruttando solo la fase di "predizione" si usano solo le misure di velocità angolare per stimare l'assetto senza le misure ulteriori della IMU
  note: I 3 metodi di stima dinamica differiscono solo per come si definisce l'innovazione, hanno infatti le stesse equazioni si meccanizzazione di base
  omega_meas : Inport
  Fase di meccanizzazione : MATLAB Function  TreatAsAtomicUnit=on
  Integrator : Integrator  InitialCondition=phi_0
  Integrator1 : Integrator  InitialCondition=theta_0
  Integrator2 : Integrator  InitialCondition=psi_0
  Integrator5 : Integrator  InitialCondition=R_0_esatta
  Meccanizzazione esatta omega misurata : MATLAB Function  TreatAsAtomicUnit=on
  cinematica inversa : MATLAB Function  TreatAsAtomicUnit=on
  phi_hat_mecc : Outport
  theta_hat_mecc : Outport  Port=2
  psi_hat_mecc : Outport  Port=3
  R_hat_mecc : Outport  Port=4
  phi_mce : Outport  Port=5
  theta_mce : Outport  Port=6
  psi_mce : Outport  Port=7
  wires:
  omega_meas/1 -> Meccanizzazione esatta omega misurata/1(omega_meas), Fase di meccanizzazione/1(omega_meas)
  Fase di meccanizzazione/1(dR_hat_mecc) -> Integrator5/1
  Integrator5/1 -> Fase di meccanizzazione/2(R_hat_mecc), R_hat_mecc/1, cinematica inversa/1(R_hat_mecc)  "R_hat_mecc"
  cinematica inversa/1(phi_hat_mecc) -> phi_hat_mecc/1
  cinematica inversa/2(theta_hat_mecc) -> theta_hat_mecc/1
  cinematica inversa/3(psi_hat_mecc) -> psi_hat_mecc/1
  Meccanizzazione esatta omega misurata/1(phi_dot) -> Integrator/1
  Meccanizzazione esatta omega misurata/2(theta_dot) -> Integrator1/1
  Meccanizzazione esatta omega misurata/3(psi_dot) -> Integrator2/1
  Integrator/1 -> phi_mce/1, Meccanizzazione esatta omega misurata/2(phi_mce)
  Integrator1/1 -> theta_mce/1, Meccanizzazione esatta omega misurata/3(theta_mce)
  Integrator2/1 -> psi_mce/1

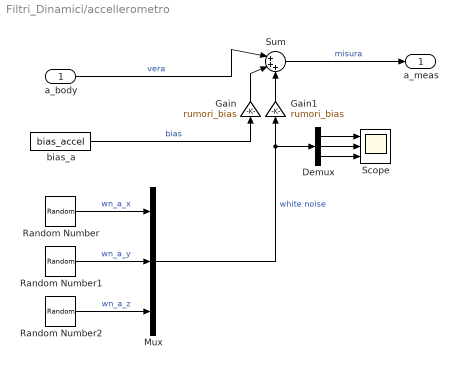
== system Filtri_Dinamici/accellerometro ==
  a_body : Inport
  Demux : Demux  Outputs=3
  Gain : Gain  Gain=rumori_bias
  Gain1 : Gain  Gain=rumori_bias
  Mux : Mux  Inputs=3
  Random Number : RandomNumber  Variance=dev_std_a_x^2  Seed=1  SampleTime=dt
  Random Number1 : RandomNumber  Variance=dev_std_a_y^2  Seed=2  SampleTime=dt
  Random Number2 : RandomNumber  Variance=dev_std_a_z^2  Seed=3  SampleTime=dt
  Scope : Scope  NumInputPorts=3
  Sum : Sum  Inputs=|+++
  bias_a : Constant  Value=bias_accel
  a_meas : Outport
  wires:
  Random Number2/1 -> Mux/3  "wn_a_z"
  bias_a/1 -> Gain/1  "bias"
  Sum/1 -> a_meas/1  "misura"
  a_body/1 -> Sum/1  "vera"
  Random Number1/1 -> Mux/2  "wn_a_y"
  Mux/1 -> Demux/1, Gain1/1  "white noise"
  Random Number/1 -> Mux/1  "wn_a_x"
  Demux/1 -> Scope/1
  Demux/2 -> Scope/2
  Demux/3 -> Scope/3
  Gain/1 -> Sum/2
  Gain1/1 -> Sum/3

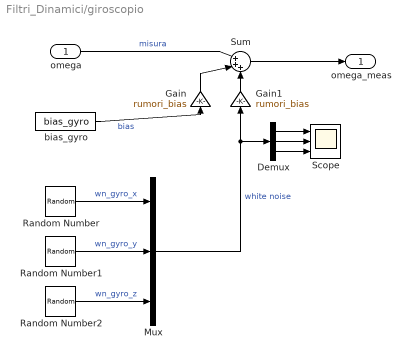
== system Filtri_Dinamici/giroscopio ==
  omega : Inport
  Demux : Demux  Outputs=3
  Gain : Gain  Gain=rumori_bias
  Gain1 : Gain  Gain=rumori_bias
  Mux : Mux  Inputs=3
  Random Number : RandomNumber  Variance=dev_std_gyro_x^2  Seed=4  SampleTime=dt
  Random Number1 : RandomNumber  Variance=dev_std_gyro_y^2  Seed=5  SampleTime=dt
  Random Number2 : RandomNumber  Variance=dev_std_gyro_z^2  Seed=6  SampleTime=dt
  Scope : Scope  NumInputPorts=3
  Sum : Sum  Inputs=|+++
  bias_gyro : Constant  Value=bias_gyro
  omega_meas : Outport
  wires:
  Sum/1 -> omega_meas/1
  omega/1 -> Sum/1  "misura"
  Demux/2 -> Scope/2
  Demux/3 -> Scope/3
  Mux/1 -> Demux/1, Gain1/1  "white noise"
  Demux/1 -> Scope/1
  Random Number2/1 -> Mux/3  "wn_gyro_z"
  Random Number/1 -> Mux/1  "wn_gyro_x"
  Random Number1/1 -> Mux/2  "wn_gyro_y"
  bias_gyro/1 -> Gain/1  "bias"
  Gain1/1 -> Sum/3
  Gain/1 -> Sum/2

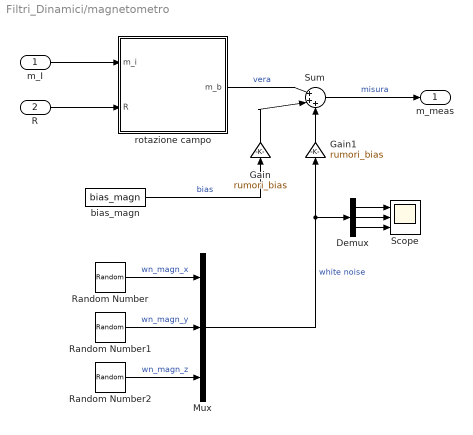
== system Filtri_Dinamici/magnetometro ==
  m_I : Inport
  R : Inport  Port=2
  Demux : Demux  Outputs=3
  Gain : Gain  Gain=rumori_bias
  Gain1 : Gain  Gain=rumori_bias
  Mux : Mux  Inputs=3
  Random Number : RandomNumber  Variance=dev_std_magn_x^2  Seed=7  SampleTime=dt
  Random Number1 : RandomNumber  Variance=dev_std_magn_y^2  Seed=8  SampleTime=dt
  Random Number2 : RandomNumber  Variance=dev_std_magn_z^2  Seed=9  SampleTime=dt
  Scope : Scope  NumInputPorts=3
  Sum : Sum  Inputs=|+++
  bias_magn : Constant  Value=bias_magn
  rotazione campo : MATLAB Function  TreatAsAtomicUnit=on
  m_meas : Outport
  wires:
  rotazione campo/1(m_b) -> Sum/1  "vera"
  R/1 -> rotazione campo/2(R)
  m_I/1 -> rotazione campo/1(m_i)
  Sum/1 -> m_meas/1  "misura"
  Demux/3 -> Scope/3
  Demux/2 -> Scope/2
  bias_magn/1 -> Gain/1  "bias"
  Random Number/1 -> Mux/1  "wn_magn_x"
  Random Number1/1 -> Mux/2  "wn_magn_y"
  Random Number2/1 -> Mux/3  "wn_magn_z"
  Demux/1 -> Scope/1
  Mux/1 -> Gain1/1, Demux/1  "white noise"
  Gain1/1 -> Sum/3
  Gain/1 -> Sum/2

== matlab function Filtri_Dinamici/cinematica inversa ==
  data: R_hat input; phi_hat output; theta_hat output; psi_hat output
function [phi_hat, theta_hat, psi_hat] = inv_kin_estim(R_hat)
% Ricavo gli angoli di Eulero stimati a partire dalla matrice di rotazione
% stimata
phi_hat = atan2(R_hat(3,2),R_hat(3,3));
theta_hat = -asin(R_hat(3,1));
psi_hat = atan2(R_hat(2,1),R_hat(1,1));

== matlab function Filtri_Dinamici/MATLAB Function ==
  data: x input; R_tilde output; dx output; m_I parameter; k1 parameter; k2 parameter; lambda output
function [R_tilde, dx, lambda] = din_err_Eulero(x, m_I, k1, k2)

% R_tilde è definito come R*R_hat';
% s = cross(k1*e3, R_hat*e3) + cross(k2*mI_bar, R_tilde*mI_bar); 
% S = [0,   -s(3),  s(2);
%      s(3),  0,   -s(1);
%     -s(2),  s(1),  0   ];
% dR_tilde = S*R_tilde;
% Linearizzando tale dinamica ottengo
mI_bar = m_I/norm(m_I);
R_tilde = eye(3) + [0,   -x(3),  x(2);
                    x(3),  0,   -x(1);
                   -x(2),  x(1),  0   ];
A = [-k1-k2*(1-mI_bar(1)^2),    k2*mI_bar(1)*mI_bar(2),   k2*mI_bar(1)*mI_bar(3);
       k2*mI_bar(1)*mI_bar(2),  -k1-k2*(1-mI_bar(2)^2),    k2*mI_bar(2)*mI_bar(3);
       k2*mI_bar(1)*mI_bar(3),   k2*mI_bar(2)*mI_bar(3),  -k2*(1-mI_bar(3)^2)     ];
dx = A* x;
% x(1) = errore di stima di roll
% x(2) = errore di stima di pitch
% x(3) = errore di stima di yaw
lambda = eig(A);
% Autovalori nel caso malcondizionato:
% lambda = [-(k1+k2);
%           -0.5*(k1+k2)*(1+sqrt(1-(4*k1*k2*mI_bar(1)^2)/(k1+k2)^2 ) );
%           -0.5*(k1+k2)*(1-sqrt(1-(4*k1*k2*mI_bar(1)^2)/(k1+k2)^2 ) )]; % autovalori della dinamica di x

== matlab function Filtri_Dinamici/Filtro di Mahony modificato da Martin e Salaun ==
  data: omega_meas input; b_omega_hat input; R_hat input; a_B input; dR_hat output; db_omega_hat output; m_B input; k1_MS parameter; k2_MS parameter; g parameter; e3 parameter; m_I parameter; k_B_MS parameter
function [dR_hat, db_omega_hat]= Martin_Salaun(omega_meas, b_omega_hat, R_hat, a_B, m_B, k1_MS, k2_MS, g, e3, m_I, k_B_MS)
% Si crea un altro vettore inerziale come il prodotto vettoriale tra la
% direzione della gravità e la direzione del campo magnetico terrestre. 
% é associato ad una misura artificiale basata sul prodotto vettoriale tra
% le misure di accellerometro e magnetometro.

% Normalizzo i vettori delle misure
uB = -a_B/g;            
uI = e3;                       
% Definizione del nuovo vettore inerziale
vI = cross(uI,m_I)/norm(cross(uI,m_I));
vB = cross(uB,m_B)/norm(cross(uB,m_B)); % ricontrollare definizione del denominatore
% Calcolo dei vettori intermedi
uB_hat = R_hat'*uI;
vB_hat = R_hat'*vI;
% Ridefinisco l'innovazione come 
sigma_R = k1_MS*cross(uB,uB_hat) + k2_MS*cross(vB,vB_hat);
% Vado ora ad applicare le equazioni del filtro complementare esplicito
sigma_b = -k_B_MS*sigma_R;  % innovazione del bias
% Calcoli intermedi
omega_inn = omega_meas-b_omega_hat+sigma_R;
S_omega_inn = [0,            -omega_inn(3),  omega_inn(2);
               omega_inn(3),    0,           -omega_inn(1);
              -omega_inn(2),  omega_inn(1),      0          ];

% Dinamica di stima della matrice di rotazione
dR_hat = R_hat*S_omega_inn;
% dinamica del bias stimato
db_omega_hat = sigma_b;

== matlab function Filtri_Dinamici/cinematica inversa1 ==
  data: R_hat input; phi_hat output; theta_hat output; psi_hat output
function [phi_hat, theta_hat, psi_hat] = inv_kin_estim(R_hat)
% Ricavo gli angoli di Eulero stimati a partire dalla matrice di rotazione
% stimata
phi_hat = atan2(R_hat(3,2),R_hat(3,3));
theta_hat = -asin(R_hat(3,1));
psi_hat = atan2(R_hat(2,1),R_hat(1,1));

== matlab function Filtri_Dinamici/Filtro di Mahony modificato (Osservatore Condizionato) ==
  data: omega_meas input; b_omega_hat input; R_hat input; a_B input; dR_hat output; db_omega_hat output; m_B input; k1_CO parameter; k2_CO parameter; g parameter; e3 parameter; m_I parameter; k3_CO parameter; k4_CO parameter; Delta parameter; kB_CO parameter
function [dR_hat, db_omega_hat]= Oss_Cond(omega_meas, b_omega_hat, R_hat, a_B, m_B, k1_CO, k2_CO, g, e3, m_I, k3_CO, k4_CO, Delta, kB_CO)
% Sempre nella forma di un filtro complementare esplicito ma con dei
% termini di innovazione definiti in maniera diversa

%========================= Calcoli preliminari ===========================%
% Normalizzo i vettori delle misure
uB = -a_B/g;    % Direzione gravitazionale misurata (-> in terna body)
uI = e3;        % Direzione gravitazionale in frame inerziale
% Calcolo le proiezioni del campo magnetico sul piano ortogonale a uI e uB
pi_uI = norm(uI)^2*eye(3) - uI*uI';
pi_uB = norm(uB)^2*eye(3) - uB*uB';
% Nuova definizione del nuovo vettore inerziale
vI = (pi_uI*m_I)/norm(pi_uI*m_I);
vB = (pi_uB*m_B)/norm(pi_uI*m_I); % ricontrollare definizione del denominatore (a ricevimento è stato detto B, su altro articolo è I)
% Calcolo dei vettori intermedi
uB_hat = R_hat' * uI;
vB_hat = R_hat' * vI;

%==================== Ridefinisco l'innovazione come =====================%
%sigma_R = k1_CO*cross(uB,uB_hat) + k2_CO* ((cross(vB,vB_hat))'*uB_hat) *uB_hat;  % innovazione della matrice di rotazione
sigma_R = k1_CO*cross(uB,uB_hat) + k2_CO*(uB_hat*uB_hat')* cross(vB,vB_hat); % innovazione della matrice di rotazione, versione di articolo di implementazione
% sigma_b = k3_CO*cross(uB,uB_hat) + k4_CO*cross(vB,vB_hat);  % innovazione del bias
sigma_b = -k3_CO*cross(uB,uB_hat) - k4_CO*cross(vB,vB_hat);  % innovazione del bias, versione articolo implementazione


%= Vado ora ad applicare le equazioni del filtro complementare esplicito =%
% Calcoli intermedi
omega_inn = omega_meas-b_omega_hat+sigma_R;
S_omega_inn = [0,            -omega_inn(3),  omega_inn(2);
               omega_inn(3),    0,           -omega_inn(1);
              -omega_inn(2),  omega_inn(1),      0          ];

% Dinamica di stima della matrice di rotazione
dR_hat = R_hat*S_omega_inn;
% dinamica del bias stimato
% db_omega_hat = sigma_b;
% dinamica del bias stimato, versione dell'articolo di implemnetazione
sat_Delta_b = b_omega_hat*min(1,Delta/norm(b_omega_hat));
db_omega_hat = -kB_CO*b_omega_hat + kB_CO*sat_Delta_b + sigma_b;

== matlab function Filtri_Dinamici/cinematica inversa2 ==
  data: R_hat input; phi_hat output; theta_hat output; psi_hat output
function [phi_hat, theta_hat, psi_hat] = inv_kin_estim(R_hat)
% Ricavo gli angoli di Eulero stimati a partire dalla matrice di rotazione
% stimata
phi_hat = atan2(R_hat(3,2),R_hat(3,3));
theta_hat = -asin(R_hat(3,1));
psi_hat = atan2(R_hat(2,1),R_hat(1,1));

== matlab function Filtri_Dinamici/check SO3 ==
  data: R_hat input; check output; detR_Mahony output
function [check, detR_Mahony] = isSO3(R_hat)
detR_Mahony = det(R_hat);
if det(R_hat) -1 <= 10^-5  % non metto det = 1 per lasciare un po di tolleranza
    check = 1;
else
    check = 0;
end

== matlab function Filtri_Dinamici/check SO3. ==
  data: R_hat input; check output; detR_MS output
function [check, detR_MS] = isSO3(R_hat)
detR_MS = det(R_hat);
if det(R_hat) -1 <= 10^-5  % non metto det = 1 per lasciare un po di tolleranza
    check = 1;
else
    check = 0;
end

== matlab function Filtri_Dinamici/check SO3, ==
  data: R_hat input; check output; detR_CO output
function [check, detR_CO] = isSO3(R_hat)
detR_CO = det(R_hat);
if det(R_hat) -1 <= 10^-5  % non metto det = 1 per lasciare un po di tolleranza
    check = 1;
else
    check = 0;
end

== matlab function Filtri_Dinamici/wrapToPi ==
  data: u input; y output
function y = wtp(u)

y = wrapToPi(u);

== matlab function Filtri_Dinamici/wrapToPi1 ==
  data: u input; y output
function y = wtp(u)

y = wrapToPi(u);

== matlab function Filtri_Dinamici/wrapToPi2 ==
  data: u input; y output
function y = wtp(u)

y = wrapToPi(u);

== matlab function Filtri_Dinamici/wtp ==
  data: u input; y output
function y = wtp(u)

y = wrapToPi(u);

== matlab function Filtri_Dinamici/wtp1 ==
  data: u input; y output
function y = wtp(u)

y = wrapToPi(u);

== matlab function Filtri_Dinamici/wtp2 ==
  data: u input; y output
function y = wtp(u)

y = wrapToPi(u);

== matlab function Filtri_Dinamici/Cinematica VTOL, impongo angoli ==
  data: t input; phi output; theta output; psi output; p_dot output; v_dot_i output; a_body output; omega output; R output; g parameter; v_inertial input; e3 parameter; Phi1 parameter; Phi2 parameter; Phi3 parameter; w_phi1 parameter; w_phi2 parameter; w_phi3 parameter; Theta1 parameter; Theta2 parameter; Theta3 parameter; w_theta1 parameter; w_theta2 parameter; w_theta3 parameter; Psi1 parameter; Psi2 parameter; Psi3 parameter; w_psi1 parameter; w_psi2 parameter; w_psi3 parameter; phi_0 parameter; theta_0 parameter; psi_0 parameter
function [phi, theta, psi, p_dot, v_dot_i, a_body, omega, R] = cinematica_esatta_ang(t,g,v_inertial,e3,Phi1, Phi2, Phi3, w_phi1, w_phi2, w_phi3, Theta1, Theta2, Theta3, w_theta1, w_theta2, w_theta3, Psi1, Psi2, Psi3, w_psi1, w_psi2, w_psi3, phi_0, theta_0, psi_0)
% vel_dot è in frame inerziale ed esatta
% v_dot_i è sempre in frame inerziale ma tiene conto dell'errore di
% integrazione numerica di Simulink

%================ Definizione traiettorie di riferimento =================%
% Moto lineare
% vel_dot = 10*[-sin(t); -2*sin(2*t); -64*cos(8*t)/128 ]; %traiettoria troppo ricca
vel_dot = zeros(3,1); % approssimazione per VTOL

% Moto angoli di Eulero
phi =   phi_0+   Phi1*sin(w_phi1*t) +     Phi2*sin(w_phi2*t) +     Phi3*sin(w_phi3*t);
theta = theta_0+ Theta1*sin(w_theta1*t) + Theta2*sin(w_theta2*t) + Theta3*sin(w_theta3*t);
psi =   psi_0 +  Psi1*sin(w_psi1*t) +     Psi2*sin(w_psi2*t) +     Psi3*sin(w_psi3*t);

% Calcolo della velocità angolare a partire dagli angoli di Eulero
dphi = Phi1*w_phi1*cos(w_phi1*t)+Phi2*w_phi2*cos(w_phi2*t)+Phi3*w_phi3*cos(w_phi3*t);
dtheta = Theta1*w_theta1*cos(w_theta1*t)+Theta2*w_theta2*cos(w_theta2*t)+Theta3*w_theta3*cos(w_theta3*t);
dpsi = Psi1*w_psi1*cos(w_psi1*t)+Psi2*w_psi2*cos(w_psi2*t)+Psi3*w_psi3*cos(w_psi3*t);
omega1 = dphi-sin(theta)*dpsi;
omega2 = cos(phi)*dtheta+cos(theta)*sin(phi)*dpsi;
omega3 = -sin(phi)*dtheta+cos(theta)*cos(phi)*dpsi;
omega = [omega1; omega2; omega3];

%================ Matrice di rotazione da body a inerziale ===============%
%(C_bi in notazione vista a lezione) esatta 
R = [cos(theta)*cos(psi),  -cos(phi)*sin(psi) + cos(psi)*sin(phi)*sin(theta),   sin(phi)*sin(psi) + cos(psi)*cos(phi)*sin(theta); 
     cos(theta)*sin(psi),   cos(phi)*cos(psi) + sin(psi)*sin(phi)*sin(theta),  -sin(phi)*cos(psi) + sin(psi)*cos(phi)*sin(theta);
     -sin(theta),           sin(phi)*cos(theta),                                cos(phi)*cos(theta)];

%============== Meccanizzazione delle velocità e posizione ===============%
% Definizione accelerazione reale in terna body
a_body = R' * (vel_dot - g*e3); 
% Inverto l'espressione per ricavarne la derivata della velocità in terna inerziale 
v_dot_i =  R*a_body + g*e3;
% Definisco la derivata della posizione come la velocità
p_dot = v_inertial;

== matlab function Filtri_Dinamici/Pura Meccanizzazione/Fase di meccanizzazione ==
  data: omega_meas input; dR_hat_mecc output; R_hat_mecc input
function dR_hat_mecc   = soloMecc(omega_meas, R_hat_mecc)
% Normalizzo i vettori delle misure
% uB = -a_B/g;            mB_bar = m_B/norm(m_I);
% uI = e3;                mI_bar = m_I/norm(m_I);   
% uB_hat = R_hat'*uI;     mB_bar_hat = R_hat'*mI_bar;

% Stavolta non calcolo le innovazioni per la matrice di rotazione e bias gyro
% sigma_R = k1*cross(uB,uB_hat) + k2*cross(mB_bar,mB_bar_hat);
% sigma_b = -k_B*sigma_R;

% Calcoli intermedi
omega_inn = omega_meas;   % -b_omega_hat +sigma_R;
S_omega_inn = [0,            -omega_inn(3),  omega_inn(2);
               omega_inn(3),    0,           -omega_inn(1);
              -omega_inn(2),  omega_inn(1),      0          ];

% Dinamica di stima della matrice di rotazione
dR_hat_mecc = R_hat_mecc*S_omega_inn;
% dinamica del bias stimato ora non compare
% db_omega_hat = sigma_b;

== matlab function Filtri_Dinamici/Pura Meccanizzazione/cinematica inversa ==
  data: R_hat_mecc input; phi_hat_mecc output; theta_hat_mecc output; psi_hat_mecc output
function [phi_hat_mecc, theta_hat_mecc, psi_hat_mecc] = inv_kin_estim(R_hat_mecc)
% Ricavo gli angoli di Eulero stimati a partire dalla matrice di rotazione
% stimata
phi_hat_mecc = atan2(R_hat_mecc(3,2),R_hat_mecc(3,3));
theta_hat_mecc = -asin(R_hat_mecc(3,1));
psi_hat_mecc = atan2(R_hat_mecc(2,1),R_hat_mecc(1,1));

== matlab function Filtri_Dinamici/Pura Meccanizzazione/Meccanizzazione esatta omega misurata ==
  data: omega_meas input; phi_dot output; phi_mce input; theta_mce input; theta_dot output; psi_dot output
function [phi_dot, theta_dot, psi_dot] = MeccEsattaCin(omega_meas, phi_mce,theta_mce)

%=================== Cinematica degli angoli di Eulero ===================%
phi_dot = omega_meas(1) + sin(phi_mce)*tan(theta_mce)*omega_meas(2) + cos(phi_mce)*tan(theta_mce)*omega_meas(3);
theta_dot = cos(phi_mce)*omega_meas(2) - sin(phi_mce)*omega_meas(3);
psi_dot = omega_meas(2)*sin(phi_mce)/cos(theta_mce) + omega_meas(3)*cos(phi_mce)/cos(theta_mce);

== matlab function Filtri_Dinamici/magnetometro/rotazione campo ==
  data: m_i input; m_b output; R input
function m_b = magn_body(m_i, R)

m_b = R'*m_i;

== matlab function Filtri_Dinamici/Cinematica VTOL, impongo omega ==
  data: t input; phi_dot output; phi input; theta input; psi input; theta_dot output; psi_dot output; p_dot output; v_dot_i output; a_body output; omega output; R output; g parameter; v_inertial input; e3 parameter; Omega12 parameter; Omega13 parameter; Omega21 parameter; Omega22 parameter; Omega23 parameter; Omega31 parameter; Omega11 parameter; Omega32 parameter; Omega33 parameter; w_11 parameter; w_12 parameter; w_13 parameter; w_21 parameter; w_22 parameter; w_23 parameter; w_31 parameter; w_32 parameter; w_33 parameter
function [phi_dot, theta_dot, psi_dot, p_dot, v_dot_i, a_body, omega, R] = cinematica_esatta(t, phi,theta,psi, g, v_inertial, e3, Omega12, Omega13, Omega21, Omega22, Omega23, Omega31, Omega11, Omega32, Omega33, w_11, w_12, w_13, w_21, w_22, w_23, w_31, w_32, w_33)
% vel_dot è in frame inerziale ed esatta
% v_dot_i è sempre in frame inerziale ma tiene conto dell'errore di
% integrazione numerica di Simulink

%================ Definizione traiettorie di riferimento =================%
% Moto lineare
% vel_dot = 10*[-sin(t); -2*sin(2*t); -64*cos(8*t)/128 ]; %traiettoria troppo ricca
vel_dot = zeros(3,1); % approssimazione per VTOL
% vel_dot = g/8*[-sin(t); -2*sin(2*t); -64*cos(8*t)/128];  % prova traiettoria lenta

% Moto angolare
omega1 = Omega11*sin(w_11*t) + Omega12*sin(w_12*t) + Omega13*sin(w_13*t);
omega2 = Omega21*sin(w_21*t) + Omega22*sin(w_22*t) + Omega23*sin(w_23*t);
omega3 = Omega31*sin(w_31*t) + Omega32*sin(w_32*t) + Omega33*sin(w_33*t);
omega = [omega1; omega2; omega3];
% omega = zeros(3,1);  % approssimazione per controllare le equazioni

%=================== Cinematica degli angoli di Eulero ===================%
phi_dot = omega(1) + sin(phi)*tan(theta)*omega(2) + cos(phi)*tan(theta)*omega(3);
theta_dot = cos(phi)*omega(2) - sin(phi)*omega(3);
psi_dot = omega(2)*sin(phi)/cos(theta) + omega(3)*cos(phi)/cos(theta);

%=============== Matrice di rotazione da body a inerziale =============== %
% (C_bi in notazione vista a lezione) esatta
R = [cos(theta)*cos(psi),  -cos(phi)*sin(psi) + cos(psi)*sin(phi)*sin(theta),   sin(phi)*sin(psi) + cos(psi)*cos(phi)*sin(theta); 
     cos(theta)*sin(psi),   cos(phi)*cos(psi) + sin(psi)*sin(phi)*sin(theta),  -sin(phi)*cos(psi) + sin(psi)*cos(phi)*sin(theta);
     -sin(theta),           sin(phi)*cos(theta),                                cos(phi)*cos(theta)];

%============== Meccanizzazione delle velocità e posizione ===============%
% Definizione accelerazione reale in terna body
a_body = R' * (vel_dot - g*e3); 
% Inverto l'espressione per ricavarne la derivata della velocità in terna inerziale 
v_dot_i =  R*a_body + g*e3;
% Definisco la derivata della posizione come la velocità
p_dot = v_inertial;

== matlab function Filtri_Dinamici/Filtro Complementare Esplicito Standard (Mahony) ==
  data: omega_meas input; dR_hat output; b_omega_hat input; R_hat input; db_omega_hat output; k1 parameter; k2 parameter; a_B input; g parameter; e3 parameter; m_B input; m_I parameter; k_B parameter
function [dR_hat, db_omega_hat]  = Mahony_std(omega_meas, b_omega_hat, R_hat, k1, k2, a_B, g, e3, m_B, m_I, k_B)
% Normalizzo i vettori delle misure
uB = -a_B/g;            mB_bar = m_B/norm(m_I);
uI = e3;                mI_bar = m_I/norm(m_I);   
uB_hat = R_hat'*uI;     mB_bar_hat = R_hat'*mI_bar;
% Calcolo le innovazioni per la matrice di rotazione e bias gyro
sigma_R = k1*cross(uB,uB_hat) + k2*cross(mB_bar,mB_bar_hat);
sigma_b = -k_B*sigma_R;
% Calcoli intermedi
omega_inn = omega_meas-b_omega_hat+sigma_R;
S_omega_inn = [0,            -omega_inn(3),  omega_inn(2);
               omega_inn(3),    0,           -omega_inn(1);
              -omega_inn(2),  omega_inn(1),      0          ];

% Dinamica di stima della matrice di rotazione
dR_hat = R_hat*S_omega_inn;
% dinamica del bias stimato
db_omega_hat = sigma_b;
